simulink model "EKF_2018b"  (R2021a)
settings: Solver=ode4  StartTime=0.0  StopTime=200  FixedStep=0.02  RelTol=1e-3
libraries: commchan3 x1
settings Model: Creator=12406  LastModifiedBy=aryal
settings SolverCC: AlgebraicLoopSolver=TrustRegion

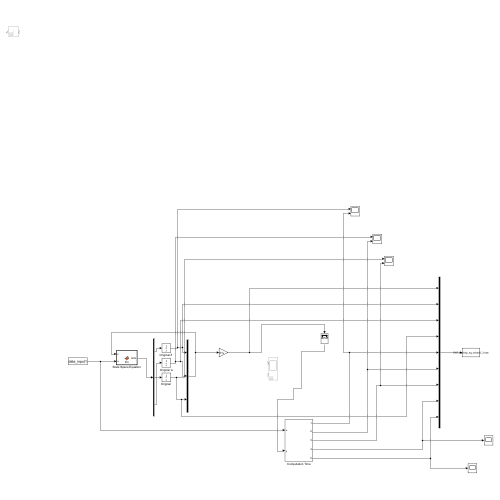
[thumbnail: Simulink's stored preview of the top-level diagram]
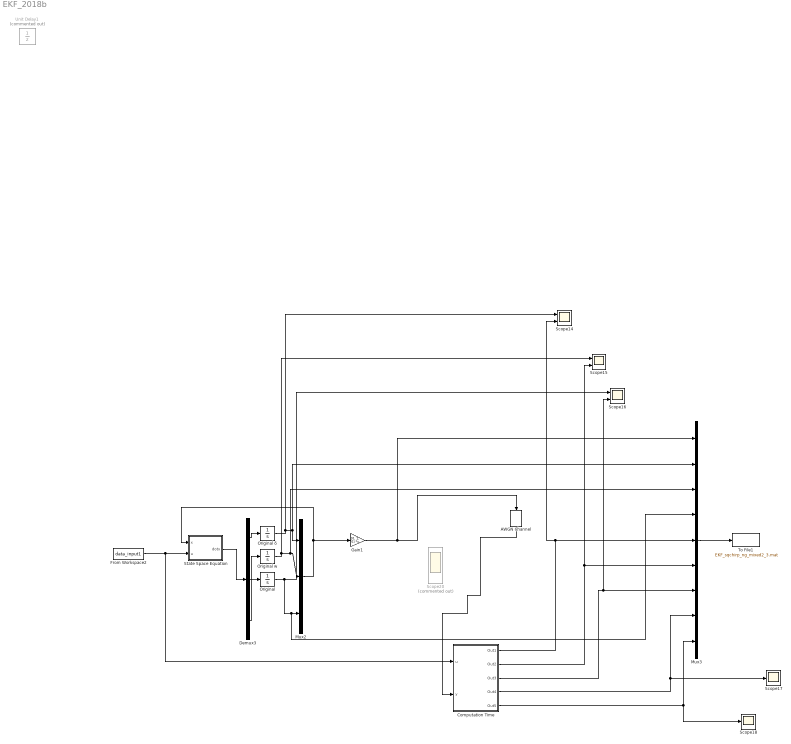
== system EKF_2018b ==
  AWGN Channel : commchan3/AWGN Channel  InputProcessing=Columns as channels (frame based)  seed=65  noiseMode=Variance from mask  EbNodB=10  EsNodB=10  SNRdB=10  bitsPerSym=1  Ps=1  Tsym=1  variance=1e-6
  Computation Time : Subsystem
  Demux3 : Demux  Outputs=3
  From Workspace2 : FromWorkspace  VariableName=data_input1  SampleTime=0.02
  Gain1 : Gain  Gain=[0, 1, 0]  Multiplication=Matrix(K*u)
  Mux2 : Mux  Inputs=3
  Mux3 : Mux  Inputs=9
  "Original " : Integrator
  Original w : Integrator
  "Original δ " : Integrator
  Scope14 : Scope  NumInputPorts=2
  Scope15 : Scope  NumInputPorts=2
  Scope16 : Scope  NumInputPorts=2
  Scope17 : Scope
  Scope18 : Scope
  Scope20 : Scope  Commented=on  NumInputPorts=2
  State Space Equation : MATLAB Function  TreatAsAtomicUnit=on
  To File1 : ToFile  Filename=EKF_sqchirp_ng_mixed2_3.mat  MatrixName=w  SampleTime=0.02
  Unit Delay1 : UnitDelay  Commented=on  InitialCondition=ones(25,1)*1e2  SampleTime=0.02  HasFrameUpgradeWarning=on
  wires:
  "Original "/1 -> Scope16/1, Mux3/4, Mux2/3
  Demux3/2 -> Original w/1
  Original w/1 -> Scope15/1, Mux3/3, Mux2/2
  "Original δ "/1 -> Scope14/1, Mux3/2, Mux2/1
  State Space Equation/1(dotx) -> Demux3/1
  From Workspace2/1 -> Computation Time/1(u), State Space Equation/2(u)
  Demux3/1 -> "Original δ "/1
  Mux2/1 -> Gain1/1, State Space Equation/1(x)
  Demux3/3 -> "Original "/1
  Gain1/1 -> AWGN Channel/1, Mux3/1
  AWGN Channel/1 -> Computation Time/2(y)
  Computation Time/1(Out1) -> Mux3/5, Scope14/2
  Computation Time/2(Out2) -> Scope15/2, Mux3/6
  Computation Time/3(Out3) -> Scope16/2, Mux3/7
  Computation Time/4(Out4) -> Scope17/1, Mux3/8
  Computation Time/5(Out5) -> Scope18/1, Mux3/9
  Mux3/1 -> To File1/1

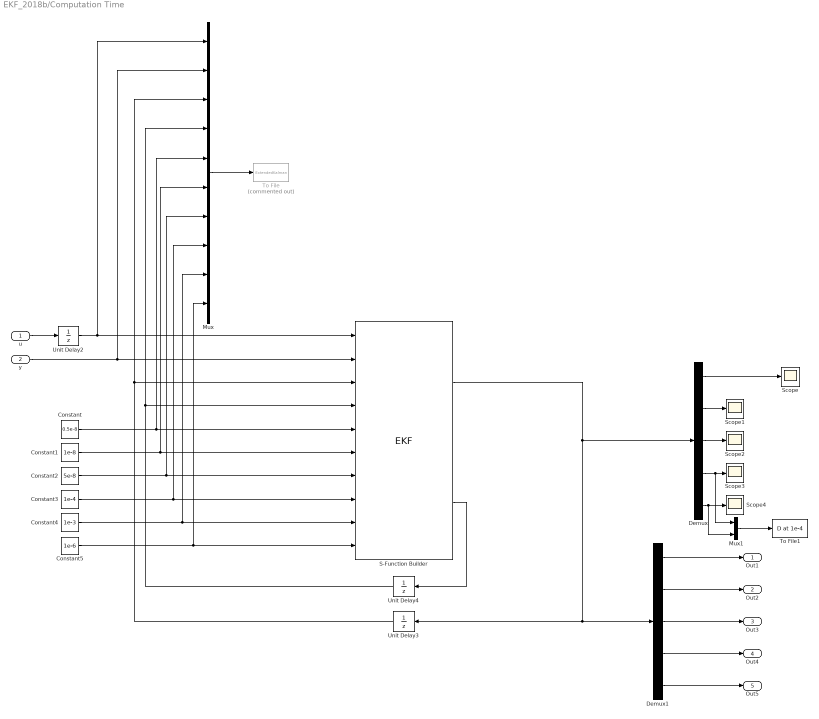
== system EKF_2018b/Computation Time ==
  u : Inport
  y : Inport  Port=2
  Constant : Constant  Value=0.5e-8
  Constant1 : Constant  Value=1e-8
  Constant2 : Constant  Value=5e-8
  Constant3 : Constant  Value=1e-4
  Constant4 : Constant  Value=1e-3
  Constant5 : Constant  Value=1e-6
  Demux : Demux  Outputs=5
  Demux1 : Demux  Outputs=5
  Mux : Mux  Inputs=10
  Mux1 : Mux  Inputs=2
  S-Function Builder : S-Function  FunctionName=EKF  SFunctionModules=EKF_wrapper EKF_Code EKF_Code_Call  SFunctionDeploymentMode=off  EnableBusSupport=off  mask(S-Function Builder){}
      mask help: Simulink:masks:SFunctionBuilder_MD
      mask init:
      | val = [[.9  0.75 0.75 1 1 .9 .9 1]',[1 1 0.75 0.75 .9 .9 1 .9]'];try , sys = get_param(gcb,'SfunBuilderFcnName');if isempty(sys), sys = get_param(gcb,'FunctionName'); end,catch, sys = get_param(gcb,'FunctionName'); end
      settings: CopyFcn=set_param(gcbh,'LinkStatus','none')  OpenFcn=sfunctionwizard(gcbh)
      mask Display: plot(val(:,1),val(:,2)),disp(sys),port_label('input',1,'u'),port_label('input',2,'y'),port_label('input',3,'xhatp'),port_label('input',4,'Pkp'),port_label('input',5,'Q11'),port_label('input',6,'Q22'),port_label('input',7,'Q33'),port_label('input',8,'Q44'),port_label('input',9,'Q55'),port_label('input',10,'R'),port_label('output',1,'xhat'),port_label('output',2,'Pk')
  Scope{,1..4} (5 alike) : Scope
  To File : ToFile  Commented=on  Filename=ExtendedKalman  SampleTime=0.02
  To File1 : ToFile  Filename=D at 1e-4  SampleTime=0.02
  Unit Delay2 : UnitDelay  SampleTime=0.02  HasFrameUpgradeWarning=on
  Unit Delay3 : UnitDelay  InitialCondition=[0;0;0;2;2]  SampleTime=0.02  HasFrameUpgradeWarning=on
  Unit Delay4 : UnitDelay  InitialCondition=reshape(diag([10, 10, 10, 10, 10]), 25, 1)  SampleTime=0.02  HasFrameUpgradeWarning=on
  Out1 : Outport
  Out2 : Outport  Port=2
  Out3 : Outport  Port=3
  Out4 : Outport  Port=4
  Out5 : Outport  Port=5
  wires:
  y/1 -> Mux/2, S-Function Builder/2
  S-Function Builder/1 -> Demux/1, Demux1/1, Unit Delay3/1
  Constant2/1 -> Mux/7, S-Function Builder/7
  u/1 -> Unit Delay2/1
  Constant4/1 -> Mux/9, S-Function Builder/9
  Unit Delay3/1 -> Mux/3, S-Function Builder/3
  Constant3/1 -> Mux/8, S-Function Builder/8
  Constant1/1 -> Mux/6, S-Function Builder/6
  Constant/1 -> Mux/5, S-Function Builder/5
  Unit Delay4/1 -> Mux/4, S-Function Builder/4
  Constant5/1 -> Mux/10, S-Function Builder/10
  Unit Delay2/1 -> Mux/1, S-Function Builder/1
  S-Function Builder/2 -> Unit Delay4/1
  Demux/1 -> Scope/1
  Demux/2 -> Scope1/1
  Demux/3 -> Scope2/1
  Demux/5 -> Mux1/2, Scope4/1
  Demux/4 -> Mux1/1, Scope3/1
  Mux/1 -> To File/1
  Demux1/2 -> Out2/1
  Demux1/1 -> Out1/1
  Demux1/3 -> Out3/1
  Demux1/4 -> Out4/1
  Demux1/5 -> Out5/1
  Mux1/1 -> To File1/1

== matlab function EKF_2018b/State Space Equation ==
  data: x input; u input; dotx output
function dotx  = fcn(x, u)
D = 1.5;
M=4;
    Tg = 0.2;
    Rp = 0.05;
    Ki=2;
    dotx = zeros(3, 1);
    x1 = x(1);
    x2 = x(2);
    x3=x(3);
    dotx = [x2;x3;-Ki/(M*Tg)*x1-(D/(M*Tg)+1/(Rp*M*Tg))*x2-(D/M+1/Tg)*x3-1/(M*Tg)*u];
